simulink model "KinematicController"  (R2017b)
settings: Solver=VariableStepAuto  StartTime=0.0  StopTime=10.0  RelTol=1e-3
values from neighbouring files (symbols this model uses):
  K1 = 5    [kinsim.m]
  K2 = 10    [kinsim.m]
  K3 = 5    [kinsim.m]
  omega_r = 1    [kinsim.m]
  R = 2    [FSMRAC_lin2.m]    (also in kinsim.m)
  v_r = 0.2    [kinsim.m]
settings Model: Creator=karam  LastModifiedBy=karam
settings DataIOCC: ReturnWorkspaceOutputs=on
settings SFSimCC: SimUseLocalCustomCode=on
settings RTWCC: RTWUseLocalCustomCode=on

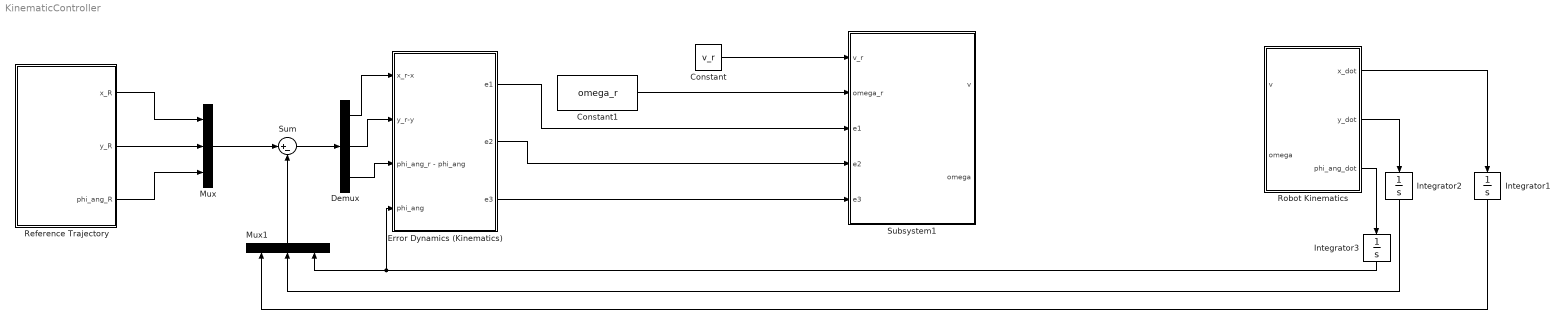
== system KinematicController ==
  Constant : Constant  Value=v_r
  Constant1 : Constant  Value=omega_r
  Demux : Demux  Outputs=3
  Error Dynamics (Kinematics) : Subsystem
  Integrator1 : Integrator
  Integrator2 : Integrator
  Integrator3 : Integrator
  Mux : Mux  Inputs=3
  Mux1 : Mux  Inputs=3
  Reference Trajectory : Subsystem
  Robot Kinematics : Subsystem
  Subsystem1 : Subsystem
  Sum : Sum  Inputs=|+-
  wires:
  Reference Trajectory/1("x_R ") -> Mux/1
  Reference Trajectory/2("y_R ") -> Mux/2
  Reference Trajectory/3("phi_ang_R ") -> Mux/3
  Mux/1 -> Sum/1
  Robot Kinematics/2(y_dot) -> Integrator2/1
  Robot Kinematics/1(x_dot) -> Integrator1/1
  Robot Kinematics/3(phi_ang_dot) -> Integrator3/1
  Integrator1/1 -> Mux1/1
  Integrator3/1 -> Mux1/3, Error Dynamics (Kinematics)/4(phi_ang)
  Integrator2/1 -> Mux1/2
  Mux1/1 -> Sum/2
  Sum/1 -> Demux/1
  Demux/1 -> Error Dynamics (Kinematics)/1("x_r-x ")
  Demux/2 -> Error Dynamics (Kinematics)/2(y_r-y)
  Demux/3 -> Error Dynamics (Kinematics)/3("phi_ang_r - phi_ang ")
  Error Dynamics (Kinematics)/1(e1) -> Subsystem1/3(e1)
  Error Dynamics (Kinematics)/2(e2) -> Subsystem1/4(e2)
  Error Dynamics (Kinematics)/3(e3) -> Subsystem1/5(e3)
  Constant/1 -> Subsystem1/1(v_r)
  Constant1/1 -> Subsystem1/2(omega_r)

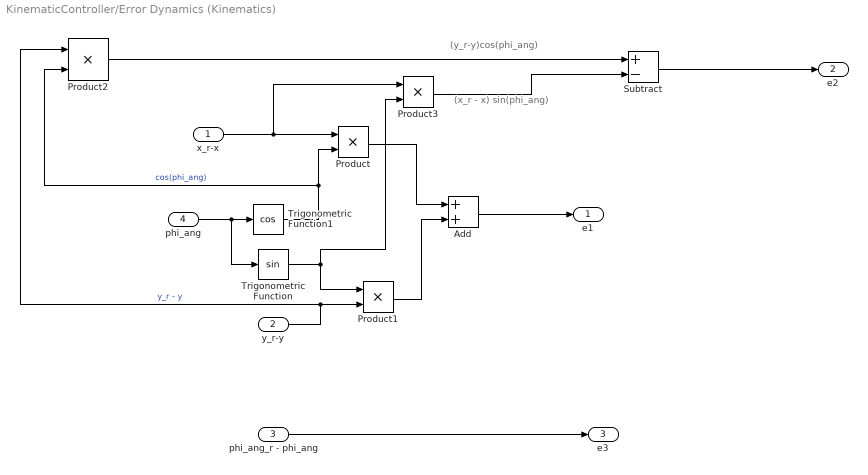
== system KinematicController/Error Dynamics (Kinematics) ==
  note: (x_r - x) sin(phi_ang)
  note: (y_r-y)cos(phi_ang)
  "x_r-x " : Inport
  y_r-y : Inport  Port=2
  "phi_ang_r - phi_ang " : Inport  Port=3
  phi_ang : Inport  Port=4
  Add : Sum
  Product{,1..3} (4 alike) : Product
  Subtract : Sum  Inputs=+-
  Trigonometric Function : Trigonometry
  Trigonometric Function1 : Trigonometry  Operator=cos
  e1 : Outport
  e2 : Outport  Port=2
  e3 : Outport  Port=3
  wires:
  "x_r-x "/1 -> Product3/1, Product/1
  phi_ang/1 -> Trigonometric Function/1, Trigonometric Function1/1
  Trigonometric Function1/1 -> Product2/2, Product/2  "cos(phi_ang)"
  Trigonometric Function/1 -> Product3/2, Product1/1
  y_r-y/1 -> Product2/1, Product1/2  "y_r - y"
  "phi_ang_r - phi_ang "/1 -> e3/1
  Product1/1 -> Add/2
  Product/1 -> Add/1
  Add/1 -> e1/1
  Product2/1 -> Subtract/1
  Product3/1 -> Subtract/2
  Subtract/1 -> e2/1

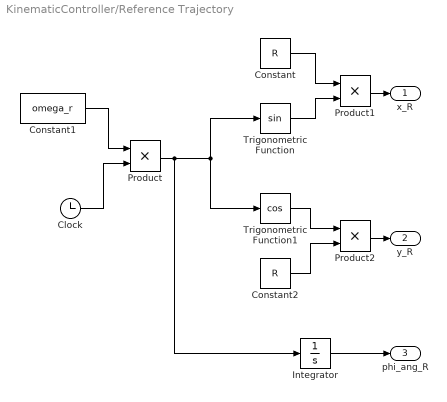
== system KinematicController/Reference Trajectory ==
  Clock : Clock
  Constant : Constant  Value=R
  Constant1 : Constant  Value=omega_r
  Constant2 : Constant  Value=R
  Integrator : Integrator
  Product : Product
  Product1 : Product
  Product2 : Product
  Trigonometric Function : Trigonometry
  Trigonometric Function1 : Trigonometry  Operator=cos
  "x_R " : Outport
  "y_R " : Outport  Port=2
  "phi_ang_R " : Outport  Port=3
  wires:
  Clock/1 -> Product/2
  Trigonometric Function1/1 -> Product2/1
  Product2/1 -> "y_R "/1
  Product/1 -> Integrator/1, Trigonometric Function1/1, Trigonometric Function/1
  Constant/1 -> Product1/1
  Product1/1 -> "x_R "/1
  Constant2/1 -> Product2/2
  Trigonometric Function/1 -> Product1/2
  Constant1/1 -> Product/1
  Integrator/1 -> "phi_ang_R "/1

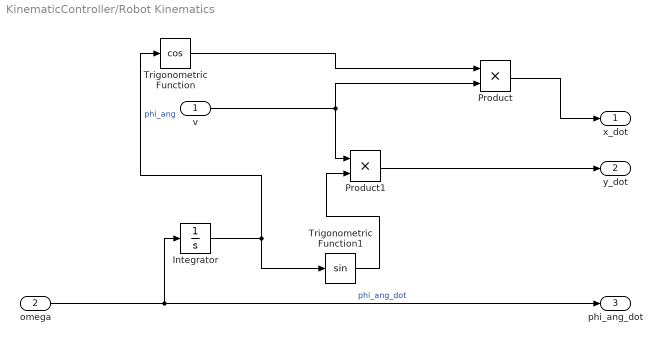
== system KinematicController/Robot Kinematics ==
  v : Inport
  omega : Inport  Port=2
  Integrator : Integrator
  Product : Product
  Product1 : Product
  Trigonometric Function : Trigonometry  Operator=cos
  Trigonometric Function1 : Trigonometry
  x_dot : Outport
  y_dot : Outport  Port=2
  phi_ang_dot : Outport  Port=3
  wires:
  omega/1 -> phi_ang_dot/1, Integrator/1  "phi_ang_dot"
  v/1 -> Product1/1, Product/2
  Integrator/1 -> Trigonometric Function/1, Trigonometric Function1/1  "phi_ang"
  Product/1 -> x_dot/1
  Trigonometric Function1/1 -> Product1/2
  Trigonometric Function/1 -> Product/1
  Product1/1 -> y_dot/1

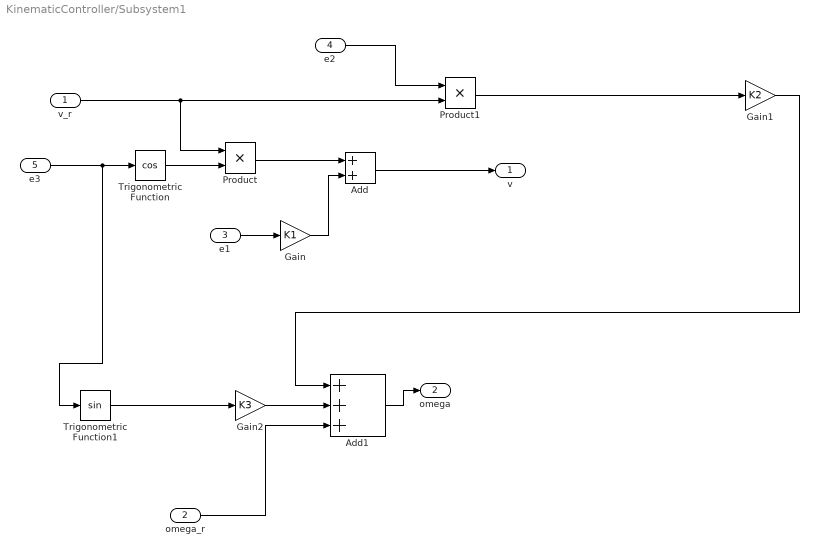
== system KinematicController/Subsystem1 ==
  v_r : Inport
  omega_r : Inport  Port=2
  e1 : Inport  Port=3
  e2 : Inport  Port=4
  e3 : Inport  Port=5
  Add : Sum
  Add1 : Sum  Inputs=+++
  Gain : Gain  Gain=K1
  Gain1 : Gain  Gain=K2
  Gain2 : Gain  Gain=K3
  Product : Product
  Product1 : Product
  Trigonometric Function : Trigonometry  Operator=cos
  Trigonometric Function1 : Trigonometry
  v : Outport
  omega : Outport  Port=2
  wires:
  Trigonometric Function/1 -> Product/2
  v_r/1 -> Product/1, Product1/2
  Product/1 -> Add/1
  e1/1 -> Gain/1
  Gain/1 -> Add/2
  Add/1 -> v/1
  Add1/1 -> omega/1
  Trigonometric Function1/1 -> Gain2/1
  e3/1 -> Trigonometric Function1/1, Trigonometric Function/1
  omega_r/1 -> Add1/3
  Gain2/1 -> Add1/2
  Gain1/1 -> Add1/1
  e2/1 -> Product1/1
  Product1/1 -> Gain1/1
